simulink library "LumAerospaceBlockset_Controllers"  (R2021a)
settings: Solver=ode45  StartTime=0.0  StopTime=10.0  RelTol=1e-3  EnableMultiTasking=on
libraries: LumAerospaceBlockset_Utilities x2, spsEdgeDetectorLib x1
settings Model: Creator=Christopher  LastModifiedBy=chris
settings SolverCC: AlgebraicLoopSolver=TrustRegion
settings DataIOCC: LimitDataPoints=on  SaveFormat=Array  ReturnWorkspaceOutputs=off
settings OptimizationCC: LifeSpan=inf
settings DebuggingCC: SolverPrmCheckMsg=warning  SFUnexpectedBacktrackingDiag=warning  SFNoUnconditionalDefaultTransitionDiag=warning  SFExecutionAtInitializationDiag=none  SFMachineParentedDataDiag=warning  ArithmeticOperatorsInVariantConditions=warning
settings HardwareCC: ProdBitPerPointer=32  ProdBitPerSizeT=32  ProdBitPerPtrDiffT=32  ProdLargestAtomicFloat=None  ProdIntDivRoundTo=Undefined  ProdEndianess=Unspecified  ProdWordSize=32  ProdHWDeviceType=32-bit Generic
settings ModelReferenceCC: PropagateSignalLabelsOutOfModel=off
settings SFSimCC: SimUseLocalCustomCode=off  CustomCodeUndefinedFunction=UseInterfaceOnly
settings RTWCC: RTWUseLocalCustomCode=off
settings CodeAppCC: StateflowObjectComments=on
settings GRTTargetCC: TargetLangStandard=C89/C90 (ANSI)
settings ConfigComp: CovMetricSettings=dw  CovSaveCumulativeToWorkspaceVar=on  CovSaveSingleToWorkspaceVar=on  CovExternalEMLEnable=off  CovSFcnEnable=off

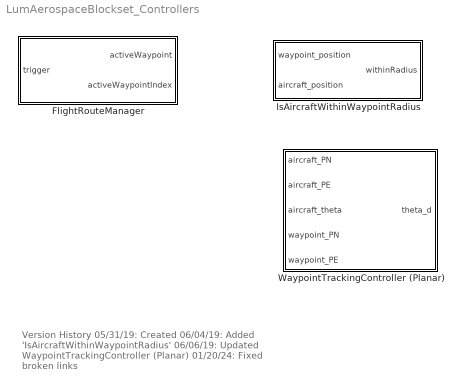
== system LumAerospaceBlockset_Controllers ==
  note: Version History
      | 05/31/19: Created
      | 06/04/19: Added 'IsAircraftWithinWaypointRadius'
      | 06/06/19: Updated WaypointTrackingController (Planar)
      | 01/20/24: Fixed broken links
  FlightRouteManager : Subsystem  mask{waypoints=0, isClosedRoute=on}
      mask prompts: waypoints "Waypoints (3xN matrix)"; isClosedRoute "Closed route"
      mask help:
      | Manages a flight route.  The flight route is a matrix of waypoints as a 3xN matrix.  This block outputs the coordinates and index of the active/current waypoint.
      |
      | When it is desired to increment the active waypoint index (for example the vehicle reaches the active/current waypoint), the 'trigger' signal should go from zero to any non-zero value to indicate this transition.  The increment of active waypoint will occur on this raising/falling edge.
      |
      | PARAMETERS:
      | -Waypoints: 3xN matrix describing the coordinates of each waypoint
      | -Closed route: checked = closed route implies that the active waypoint after the last waypoint is the first waypoint (wraps around), unchecked = open route and the active waypoint will remain at the last waypoint.
      |
      | INPUT:
      | -trigger: triggering signal
      |
      | OUTPUT:
      | -activeWaypoint:	3x1 coordinate of the active waypoint
      | -activeWaypointIndex:	active waypoint index
      |
      | Created by Christopher Lum
      | lum@uw.edu
  IsAircraftWithinWaypointRadius : Subsystem  mask{R=0}
      mask prompts: R "Waypoint radius"
      mask help:
      | Simple logic to determine if a vehicle has reached within a certain radius of a waypoint.
      |
      | PARAMETERS:
      | -Waypoint radius: waypoint is reached when vehicle is within this distance of the waypoint
      |
      | INPUT:
      | -waypoint_position: 3 element vector describing the position of the waypoint
      | -aircraft_position: 3 element vector describing the position of the aircraft
      |
      | OUTPUT:
      | -withinRadius: boolean denoting if aircraft is within radius or not.
      |
      | Created by Christopher Lum
      | lum@uw.edu
      mask TypeOptions R: Constant/Value
  WaypointTrackingController (Planar) : Subsystem
      mask help:
      | Determine the heading angle the aircraft should have in order to be pointing towards the waypoint.
      |
      | PARAMETERS:
      | -None
      |
      | INPUT:
      | -aircraft_PN: position north of the aircraft
      | -aircraft_PE: position east of the aircraft
      | -aircraft_theta: heading angle of the aircraft (0 = pointing East, positive CCW)
      | -waypoint_PN: position north of the waypoint
      | -waypoint_PE: position east of the waypoint
      |
      | OUTPUT:
      | -theta_d: desired heading angle so aircraft is pointing towards waypoint
      |
      | Created by Christopher Lum
      | lum@uw.edu

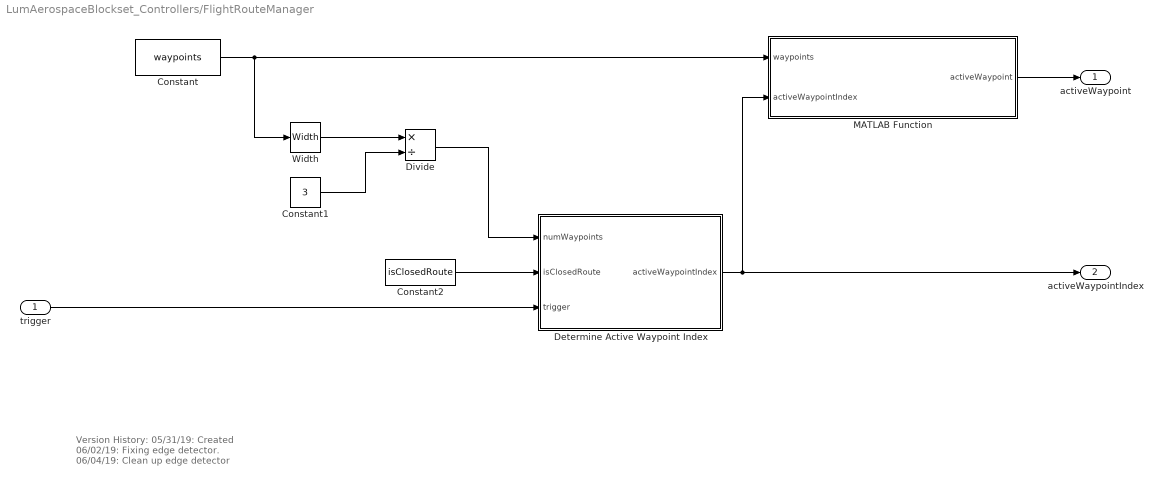
== system LumAerospaceBlockset_Controllers/FlightRouteManager ==
  note: Version History:
      | 05/31/19: Created
      | 06/02/19: Fixing edge detector.
      | 06/04/19: Clean up edge detector
  trigger : Inport
  Constant : Constant  Value=waypoints
  Constant1 : Constant  Value=3
  Constant2 : Constant  Value=isClosedRoute  OutDataTypeStr=boolean
  Determine Active Waypoint Index : Subsystem
  Divide : Product  Inputs=*/
  MATLAB Function : MATLAB Function  TreatAsAtomicUnit=on
  Width : Width
  activeWaypoint : Outport  VectorParamsAs1DForOutWhenUnconnected=off
  activeWaypointIndex : Outport  Port=2  VectorParamsAs1DForOutWhenUnconnected=off
  wires:
  Constant/1 -> Width/1, MATLAB Function/1(waypoints)
  MATLAB Function/1(activeWaypoint) -> activeWaypoint/1
  Determine Active Waypoint Index/1(activeWaypointIndex) -> MATLAB Function/2(activeWaypointIndex), activeWaypointIndex/1
  Width/1 -> Divide/1
  Constant1/1 -> Divide/2
  Divide/1 -> Determine Active Waypoint Index/1(numWaypoints)
  trigger/1 -> Determine Active Waypoint Index/3(trigger)
  Constant2/1 -> Determine Active Waypoint Index/2(isClosedRoute)

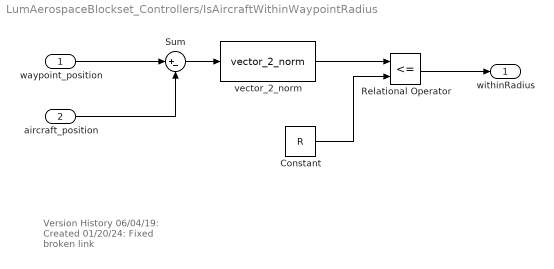
== system LumAerospaceBlockset_Controllers/IsAircraftWithinWaypointRadius ==
  note: Version History
      | 06/04/19: Created
      | 01/20/24: Fixed broken link
  waypoint_position : Inport
  aircraft_position : Inport  Port=2
  Constant : Constant  Value=R
  Relational Operator : RelationalOperator  Operator=<=  OutDataTypeStr=boolean  RndMeth=Simplest
  Sum : Sum  Inputs=|+-
  vector_2_norm : LumAerospaceBlockset_Utilities/vector_2_norm
  withinRadius : Outport  VectorParamsAs1DForOutWhenUnconnected=off
  wires:
  waypoint_position/1 -> Sum/1
  aircraft_position/1 -> Sum/2
  Sum/1 -> vector_2_norm/1
  vector_2_norm/1 -> Relational Operator/1
  Constant/1 -> Relational Operator/2
  Relational Operator/1 -> withinRadius/1

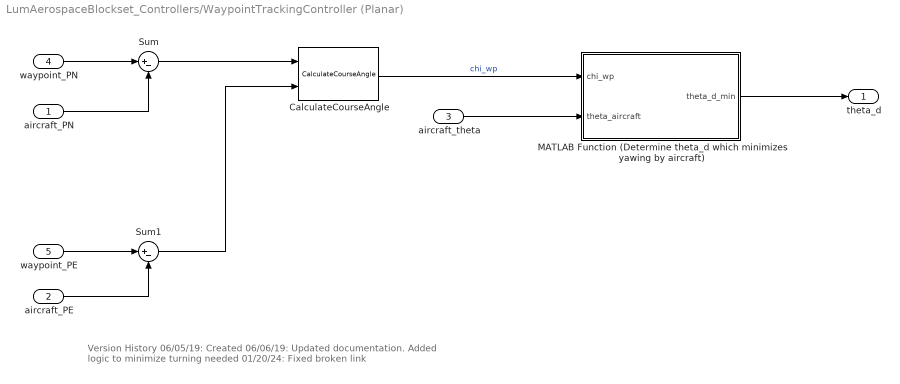
== system LumAerospaceBlockset_Controllers/WaypointTrackingController (Planar) ==
  note: Version History
      | 06/05/19: Created
      | 06/06/19: Updated documentation.  Added logic to minimize turning needed
      | 01/20/24: Fixed broken link
  aircraft_PN : Inport
  aircraft_PE : Inport  Port=2
  aircraft_theta : Inport  Port=3
  waypoint_PN : Inport  Port=4
  waypoint_PE : Inport  Port=5
  CalculateCourseAngle : LumAerospaceBlockset_Utilities/CalculateCourseAngle
  MATLAB Function (Determine theta_d which minimizes yawing by aircraft) : MATLAB Function  TreatAsAtomicUnit=on
  Sum : Sum  Inputs=|+-
  Sum1 : Sum  Inputs=|+-
  theta_d : Outport  VectorParamsAs1DForOutWhenUnconnected=off
  wires:
  waypoint_PN/1 -> Sum/1
  aircraft_PN/1 -> Sum/2
  waypoint_PE/1 -> Sum1/1
  aircraft_PE/1 -> Sum1/2
  Sum/1 -> CalculateCourseAngle/1
  Sum1/1 -> CalculateCourseAngle/2
  CalculateCourseAngle/1 -> MATLAB Function (Determine theta_d which minimizes yawing by aircraft)/1(chi_wp)  "chi_wp"
  aircraft_theta/1 -> MATLAB Function (Determine theta_d which minimizes yawing by aircraft)/2(theta_aircraft)
  MATLAB Function (Determine theta_d which minimizes yawing by aircraft)/1(theta_d_min) -> theta_d/1

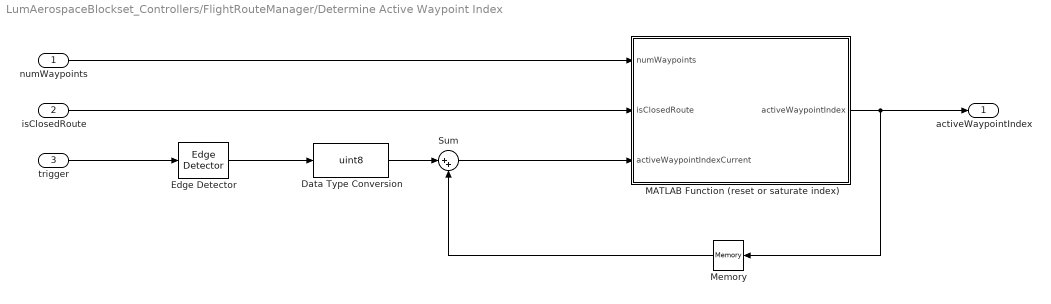
== system LumAerospaceBlockset_Controllers/FlightRouteManager/Determine Active Waypoint Index ==
  numWaypoints : Inport
  isClosedRoute : Inport  Port=2
  trigger : Inport  Port=3
  Data Type Conversion : DataTypeConversion  OutDataTypeStr=uint8
  Edge Detector : spsEdgeDetectorLib/Edge Detector  model=Rising  ic=0  Ts=0
      settings: SourceProductBaseCode=PS
  MATLAB Function (reset or saturate index) : MATLAB Function  TreatAsAtomicUnit=on
  Memory : Memory  InitialCondition=1
  Sum : Sum  Inputs=|++
  activeWaypointIndex : Outport  VectorParamsAs1DForOutWhenUnconnected=off
  wires:
  Data Type Conversion/1 -> Sum/1
  Edge Detector/1 -> Data Type Conversion/1
  Memory/1 -> Sum/2
  Sum/1 -> MATLAB Function (reset or saturate index)/3(activeWaypointIndexCurrent)
  numWaypoints/1 -> MATLAB Function (reset or saturate index)/1(numWaypoints)
  MATLAB Function (reset or saturate index)/1(activeWaypointIndex) -> Memory/1, activeWaypointIndex/1
  trigger/1 -> Edge Detector/1
  isClosedRoute/1 -> MATLAB Function (reset or saturate index)/2(isClosedRoute)

== matlab function LumAerospaceBlockset_Controllers/FlightRouteManager/MATLAB Function ==
  data: waypoints input; activeWaypoint output; activeWaypointIndex input
function activeWaypoint = fcn(waypoints, activeWaypointIndex)

%Create a FlightRoute object
flightRoute = FlightRoute(waypoints);

activeWaypoint = flightRoute.GetPoint(activeWaypointIndex);

== matlab function LumAerospaceBlockset_Controllers/WaypointTrackingController (Planar)/MATLAB Function (Determine theta_d which minimizes yawing by aircraft) ==
  data: chi_wp input; theta_d_min output; theta_aircraft input
function theta_d_min  = fcn(chi_wp, theta_aircraft)

%convert chi to theta
theta_d = pi/2 - chi_wp;

%Determine if we need to add or subtract 2*pi to minimize required turning
theta_d_p2p = theta_d + 2*pi;
theta_d_m2p = theta_d - 2*pi;

%which yields the least error between the current aircraft theta
e_theta = theta_d - theta_aircraft;
e_theta_p2p = theta_d_p2p - theta_aircraft;
e_theta_m2p = theta_d_m2p - theta_aircraft;

[~,index] = min(abs([e_theta e_theta_p2p e_theta_m2p]));

switch index
    case 1
        %theta_d is best
        theta_d_min = theta_d;
        
    case 2
        %theta_d_p2p is best
        theta_d_min = theta_d_p2p;
        
    case 3
        %theta_d_m2p is best
        theta_d_min = e_theta_m2p;
        
    otherwise
        error('Unexpected error')
end

== matlab function LumAerospaceBlockset_Controllers/FlightRouteManager/Determine Active Waypoint Index/MATLAB Function (reset or saturate index) ==
  data: numWaypoints input; isClosedRoute input; activeWaypointIndex output; activeWaypointIndexCurrent input
function activeWaypointIndex = fcn(numWaypoints, isClosedRoute, activeWaypointIndexCurrent)

%Saturate at maximum limit
if(activeWaypointIndexCurrent > numWaypoints)
    if(isClosedRoute)
        %Closed route: restart at waypoint 1
        activeWaypointIndex = 1;
    else
        %Open route: staturate at last waypoint.
        activeWaypointIndex = numWaypoints;
    end
    
else
    activeWaypointIndex = activeWaypointIndexCurrent;
    
end
